simulink model "Q8_SIM"  (R2024b)
settings: Solver=VariableStepAuto  StartTime=0.0  StopTime=10.0  RelTol=1e-3
values from neighbouring files (symbols this model uses):
  D = zeros(2,1)    [main.m]
  K = lqr(A, B, Qr, Rr)    [IP_MACRO.m]    (also in main_sim.m = lqr(A_aug, B_aug, Qr, Rr))
  L = lqe(A, G, C, Qe, Re)    [IP_MACRO.m]    (also in main.m; main_sim.m)
  x0 = [alpha_init 0 beta_init 0 0]'    [main.m]    (also in main_sim.m = [alpha_init 0 beta_init 0 0])
undefined symbols (not defined in the file or in its folder): A, B, C
settings Model: Creator=pedro  LastModifiedBy=pedro

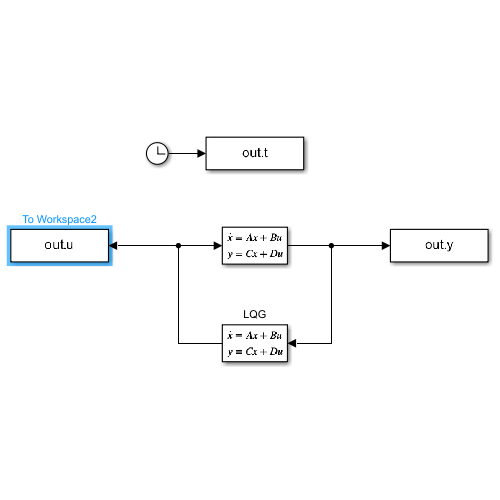
[thumbnail: Simulink's stored preview of the top-level diagram]
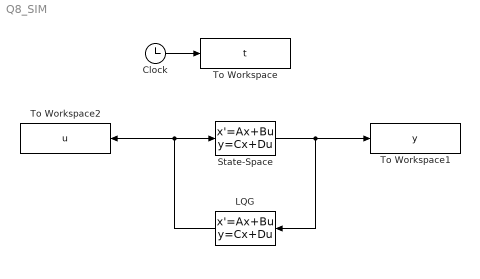
== system Q8_SIM ==
  Clock : Clock
  LQG : StateSpace  A=A - B * K - L * C  B=L  C=-K  D=zeros(1,2)  InitialCondition=0
  State-Space : StateSpace  A=A  B=B  C=C  D=D  InitialCondition=x0
  To Workspace : ToWorkspace  VariableName=t  SaveFormat=Timeseries  SampleTime=-1
  To Workspace1 : ToWorkspace  VariableName=y  SaveFormat=Timeseries  SampleTime=-1
  To Workspace2 : ToWorkspace  VariableName=u  SaveFormat=Timeseries  SampleTime=-1
  wires:
  Clock/1 -> To Workspace/1
  LQG/1 -> To Workspace2/1, State-Space/1
  State-Space/1 -> To Workspace1/1, LQG/1
